simulink library "MickLibBlocks"  (R2014a)
settings: Solver=ode45  StartTime=0.0  StopTime=10.0  RelTol=1e-3
values from neighbouring files (symbols this model uses):
  a = param.a    [DSC_Control_Analysis.m]    (also in DSC_Control_Analysis_Exp.m; DSC_Speed_Control_Analysis.m; EmpiricalTireCurves.m = 1.35; FFW_Fx.m = sqrt(curvature/(2*clothoidLength)))
  b = 1.15    [EmpiricalTireCurves.m]
  Cf = param.fl.C + param.fr.C    [Fyf_lookup_table.m]
  FFWax = fliplr(ax)    [FFW_Fx.m]
  m = 1724    [EmpiricalTireCurves.m]
  max_axRegen = -90*2*.91*5.5/.32/m    [FFW_Fx.m]
  maxUxRegen = max(UxRegen)    [FFW_Fx.m]
  s = 0:Step:round(sMax/Step)*Step    [FFW_Fx.m]
  Ts = 0.002    [DSC_Control_Analysis.m]    (also in DSC_Control_Analysis_Exp.m; DSC_Speed_Control_Analysis.m; EC_params_nissan.m; Ext_MPCPara.m = SSD.Ts)
  UxConstant = sqrt(mu*trackRadius*g)    [FFW_Fx.m]
undefined symbols (not defined in the file or in its folder): alphaFrontLimit, alphaRearLimit, Cr, filtera, filterb, gain_force_psi, gainFrontAlphaSlip, gainRearAlphaSlip, gainRearKappaSlip, gainRearNoneSlip, kappaFrontLimit, kappaRearLimit, lkparams, numberFIR_force, param, psi_threshold, sr, steering_limit, wc
libraries: UserBlocks x6, simulink_need_slupdate x3, MickLibBlocks x2
(part 1 of 2)
settings Model: Creator=ddl  LastModifiedBy=cbeal

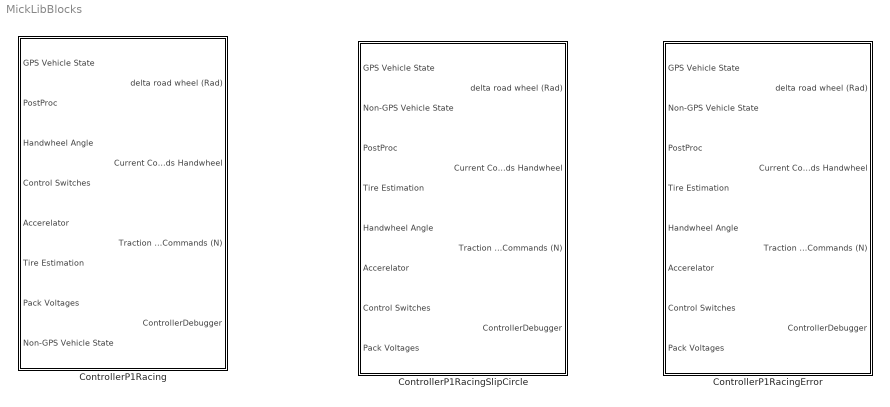
== system MickLibBlocks ==
  ControllerP1Racing : Subsystem
      mask init:
      | p1_params
  ControllerP1RacingError : Subsystem
      mask init:
      | p1_params
  ControllerP1RacingSlipCircle : Subsystem
      mask init:
      | p1_params

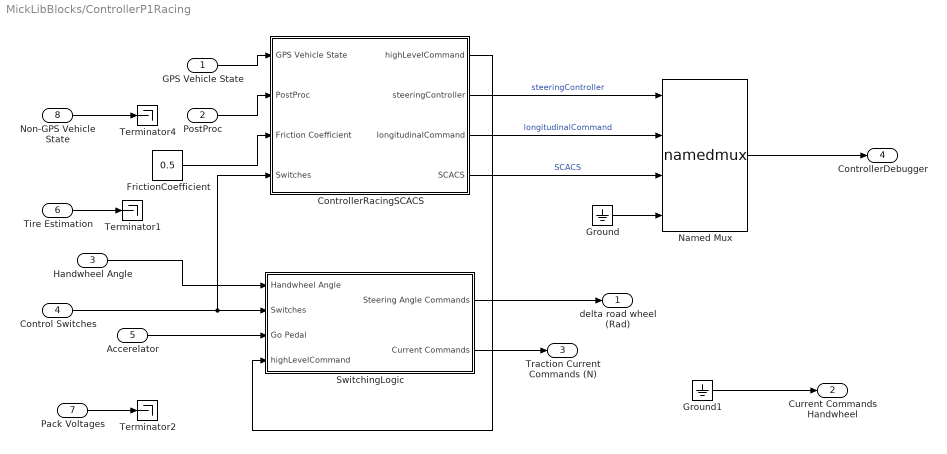
== system MickLibBlocks/ControllerP1Racing ==
  GPS Vehicle State : Inport
  PostProc : Inport  Port=2
  Handwheel Angle : Inport  Port=3
  Control Switches : Inport  Port=4
  Accerelator : Inport  Port=5
  Tire Estimation : Inport  Port=6
  Pack Voltages : Inport  Port=7
  Non-GPS Vehicle State : Inport  Port=8
  ControllerRacingSCACS : Subsystem
      mask init:
      | p1_params
  FrictionCoefficient : Constant  Value=0.5
  Ground : Ground
  Ground1 : Ground
  Named Mux : S-Function  FunctionName=namedmux  Parameters=inputcount,inputsizes  EnableBusSupport=off  mask{fname=datadescRacing}
      mask prompts: fname "Data description function name"
      mask help:
      | Combines input signals into a single output vector, according to a structure that provides the names and sizes of each signal.
      |
      | The parameter below should be set to the name of a function which returns a 1xN structure array, where N is the number of input signals.  The structure should contain fields "size" which specifies the width of the input signal, and "name" which specifies its name.
      mask init:
      | desc=eval(fname);
      | %if(class(desc)~='cell')
      | %	error('Incorrect description');
      | %end
      | inputcount=length(desc);
      | if((inputcount<1)|(inputcount>50))
      | 	error('Inappropriate number of inputs.');
      | end
      | 
      | inputsizes=[desc.size];
      | 
      | x=min(inputcount*ones(1,50),1:50);
      mask Display:
      | port_label('input',x(1),desc(x(1)).name);
      | port_label('input',x(2),desc(x(2)).name);
      | port_label('input',x(3),desc(x(3)).name);
      | port_label('input',x(4),desc(x(4)).name);
      | port_label('input',x(5),desc(x(5)).name);
      | port_label('input',x(6),desc(x(6)).name);
      | port_label('input',x(7),desc(x(7)).name);
      | port_label('input',x(8),desc(x(8)).name);
      | port_label('input',x(9),desc(x(9)).name);
      | port_label('input',x(10),desc(x(10)).name);
      | port_label('input',x(11),desc(x(11)).name);
      | port_label('input',x(12),desc(x(12)).name);
      | port_label('input',x(13),desc(x(13)).name);
      | port_label('input',x(14),desc(x(14)).name);
      | port_label('input',x(15),desc(x(15)).name);
      | port_label('input',x(16),desc(x(16)).name);
      | port_label('input',x(17),desc(x(17)).name);
      | port_label('input',x(18),desc(x(18)).name);
      | port_label('input',x(19),desc(x(19)).name);
      | port_label('input',x(20),desc(x(20)).name);
      | port_label('input',x(21),desc(x(21)).name);
      | port_label('input',x(22),desc(x(22)).name);
      | port_label('input',x(23),desc(x(23)).name);
      | port_label('input',x(24),desc(x(24)).name);
      | port_label('input',x(25),desc(x(25)).name);
      | port_label('input',x(26),desc(x(26)).name);
      | port_label('input',x(27),desc(x(27)).name);
      | port_label('input',x(28),desc(x(28)).name);
      | port_label('input',x(29),desc(x(29)).name);
      | port_label('input',x(30),desc(x(30)).name);
  SwitchingLogic : Subsystem
      mask init:
      | p1_params;
      | SteeringController;
  Terminator1 : Terminator
  Terminator2 : Terminator
  Terminator4 : Terminator
  delta road wheel (Rad) : Outport
  Current Commands Handwheel : Outport  Port=2
  Traction Current Commands (N) : Outport  Port=3
  ControllerDebugger : Outport  Port=4
  wires:
  Ground1/1 -> Current Commands Handwheel/1
  Named Mux/1 -> ControllerDebugger/1
  ControllerRacingSCACS/1(highLevelCommand) -> SwitchingLogic/4(highLevelCommand)
  GPS Vehicle State/1 -> ControllerRacingSCACS/1(GPS Vehicle State)
  PostProc/1 -> ControllerRacingSCACS/2(PostProc)
  Handwheel Angle/1 -> SwitchingLogic/1(Handwheel Angle)
  Accerelator/1 -> SwitchingLogic/3(Go Pedal)
  Control Switches/1 -> ControllerRacingSCACS/4(Switches), SwitchingLogic/2(Switches)
  SwitchingLogic/1(Steering Angle Commands) -> delta road wheel (Rad)/1
  SwitchingLogic/2(Current Commands) -> Traction Current Commands (N)/1
  ControllerRacingSCACS/2(steeringController) -> Named Mux/1  "steeringController"
  ControllerRacingSCACS/3(longitudinalCommand) -> Named Mux/2  "longitudinalCommand"
  ControllerRacingSCACS/4(SCACS) -> Named Mux/3  "SCACS"
  Non-GPS Vehicle State/1 -> Terminator4/1
  Tire Estimation/1 -> Terminator1/1
  Pack Voltages/1 -> Terminator2/1
  FrictionCoefficient/1 -> ControllerRacingSCACS/3(Friction Coefficient)
  Ground/1 -> Named Mux/4

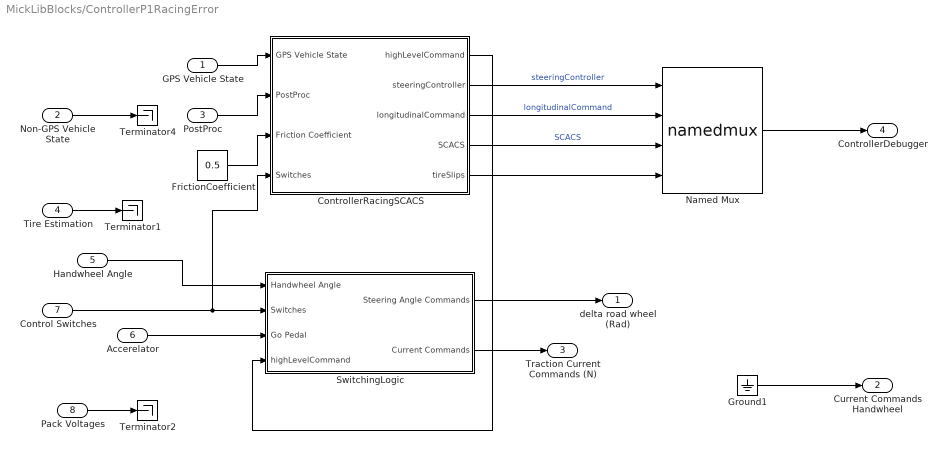
== system MickLibBlocks/ControllerP1RacingError ==
  GPS Vehicle State : Inport
  Non-GPS Vehicle State : Inport  Port=2
  PostProc : Inport  Port=3
  Tire Estimation : Inport  Port=4
  Handwheel Angle : Inport  Port=5
  Accerelator : Inport  Port=6
  Control Switches : Inport  Port=7
  Pack Voltages : Inport  Port=8
  ControllerRacingSCACS : Subsystem
      mask init:
      | p1_params
  FrictionCoefficient : Constant  Value=0.5
  Ground1 : Ground
  Named Mux : S-Function  FunctionName=namedmux  Parameters=inputcount,inputsizes  EnableBusSupport=off  mask{fname=datadescRacing}
      mask prompts: fname "Data description function name"
      mask help:
      | Combines input signals into a single output vector, according to a structure that provides the names and sizes of each signal.
      |
      | The parameter below should be set to the name of a function which returns a 1xN structure array, where N is the number of input signals.  The structure should contain fields "size" which specifies the width of the input signal, and "name" which specifies its name.
      mask init: same as MickLibBlocks/ControllerP1Racing/Named Mux
      mask Display:
      | port_label('input',x(1),desc(x(1)).name);
      | port_label('input',x(2),desc(x(2)).name);
      | port_label('input',x(3),desc(x(3)).name);
      | port_label('input',x(4),desc(x(4)).name);
      | port_label('input',x(5),desc(x(5)).name);
      | port_label('input',x(6),desc(x(6)).name);
      | port_label('input',x(7),desc(x(7)).name);
      | port_label('input',x(8),desc(x(8)).name);
      | port_label('input',x(9),desc(x(9)).name);
      | port_label('input',x(10),desc(x(10)).name);
      | port_label('input',x(11),desc(x(11)).name);
      | port_label('input',x(12),desc(x(12)).name);
      | port_label('input',x(13),desc(x(13)).name);
      | port_label('input',x(14),desc(x(14)).name);
      | port_label('input',x(15),desc(x(15)).name);
      | port_label('input',x(16),desc(x(16)).name);
      | port_label('input',x(17),desc(x(17)).name);
      | port_label('input',x(18),desc(x(18)).name);
      | port_label('input',x(19),desc(x(19)).name);
      | port_label('input',x(20),desc(x(20)).name);
      | port_label('input',x(21),desc(x(21)).name);
      | port_label('input',x(22),desc(x(22)).name);
      | port_label('input',x(23),desc(x(23)).name);
      | port_label('input',x(24),desc(x(24)).name);
      | port_label('input',x(25),desc(x(25)).name);
      | port_label('input',x(26),desc(x(26)).name);
      | port_label('input',x(27),desc(x(27)).name);
      | port_label('input',x(28),desc(x(28)).name);
      | port_label('input',x(29),desc(x(29)).name);
      | port_label('input',x(30),desc(x(30)).name);
  SwitchingLogic : Subsystem
      mask init:
      | p1_params;
      | SteeringController;
  Terminator1 : Terminator
  Terminator2 : Terminator
  Terminator4 : Terminator
  delta road wheel (Rad) : Outport
  Current Commands Handwheel : Outport  Port=2
  Traction Current Commands (N) : Outport  Port=3
  ControllerDebugger : Outport  Port=4
  wires:
  Ground1/1 -> Current Commands Handwheel/1
  FrictionCoefficient/1 -> ControllerRacingSCACS/3(Friction Coefficient)
  Pack Voltages/1 -> Terminator2/1
  Tire Estimation/1 -> Terminator1/1
  Non-GPS Vehicle State/1 -> Terminator4/1
  ControllerRacingSCACS/4(SCACS) -> Named Mux/3  "SCACS"
  ControllerRacingSCACS/3(longitudinalCommand) -> Named Mux/2  "longitudinalCommand"
  ControllerRacingSCACS/2(steeringController) -> Named Mux/1  "steeringController"
  SwitchingLogic/2(Current Commands) -> Traction Current Commands (N)/1
  SwitchingLogic/1(Steering Angle Commands) -> delta road wheel (Rad)/1
  Control Switches/1 -> SwitchingLogic/2(Switches), ControllerRacingSCACS/4(Switches)
  Accerelator/1 -> SwitchingLogic/3(Go Pedal)
  Handwheel Angle/1 -> SwitchingLogic/1(Handwheel Angle)
  PostProc/1 -> ControllerRacingSCACS/2(PostProc)
  GPS Vehicle State/1 -> ControllerRacingSCACS/1(GPS Vehicle State)
  ControllerRacingSCACS/1(highLevelCommand) -> SwitchingLogic/4(highLevelCommand)
  Named Mux/1 -> ControllerDebugger/1
  ControllerRacingSCACS/5(tireSlips) -> Named Mux/4

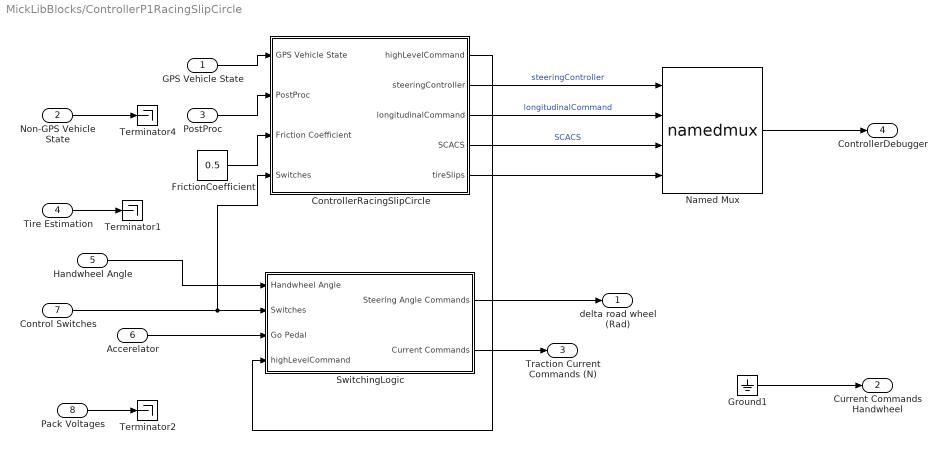
== system MickLibBlocks/ControllerP1RacingSlipCircle ==
  GPS Vehicle State : Inport
  Non-GPS Vehicle State : Inport  Port=2
  PostProc : Inport  Port=3
  Tire Estimation : Inport  Port=4
  Handwheel Angle : Inport  Port=5
  Accerelator : Inport  Port=6
  Control Switches : Inport  Port=7
  Pack Voltages : Inport  Port=8
  ControllerRacingSlipCircle : Subsystem
      mask init:
      | p1_params
  FrictionCoefficient : Constant  Value=0.5
  Ground1 : Ground
  Named Mux : S-Function  FunctionName=namedmux  Parameters=inputcount,inputsizes  EnableBusSupport=off  mask{fname=datadescRacing}
      mask prompts: fname "Data description function name"
      mask help:
      | Combines input signals into a single output vector, according to a structure that provides the names and sizes of each signal.
      |
      | The parameter below should be set to the name of a function which returns a 1xN structure array, where N is the number of input signals.  The structure should contain fields "size" which specifies the width of the input signal, and "name" which specifies its name.
      mask init: same as MickLibBlocks/ControllerP1Racing/Named Mux
      mask Display:
      | port_label('input',x(1),desc(x(1)).name);
      | port_label('input',x(2),desc(x(2)).name);
      | port_label('input',x(3),desc(x(3)).name);
      | port_label('input',x(4),desc(x(4)).name);
      | port_label('input',x(5),desc(x(5)).name);
      | port_label('input',x(6),desc(x(6)).name);
      | port_label('input',x(7),desc(x(7)).name);
      | port_label('input',x(8),desc(x(8)).name);
      | port_label('input',x(9),desc(x(9)).name);
      | port_label('input',x(10),desc(x(10)).name);
      | port_label('input',x(11),desc(x(11)).name);
      | port_label('input',x(12),desc(x(12)).name);
      | port_label('input',x(13),desc(x(13)).name);
      | port_label('input',x(14),desc(x(14)).name);
      | port_label('input',x(15),desc(x(15)).name);
      | port_label('input',x(16),desc(x(16)).name);
      | port_label('input',x(17),desc(x(17)).name);
      | port_label('input',x(18),desc(x(18)).name);
      | port_label('input',x(19),desc(x(19)).name);
      | port_label('input',x(20),desc(x(20)).name);
      | port_label('input',x(21),desc(x(21)).name);
      | port_label('input',x(22),desc(x(22)).name);
      | port_label('input',x(23),desc(x(23)).name);
      | port_label('input',x(24),desc(x(24)).name);
      | port_label('input',x(25),desc(x(25)).name);
      | port_label('input',x(26),desc(x(26)).name);
      | port_label('input',x(27),desc(x(27)).name);
      | port_label('input',x(28),desc(x(28)).name);
      | port_label('input',x(29),desc(x(29)).name);
      | port_label('input',x(30),desc(x(30)).name);
  SwitchingLogic : Subsystem
      mask init:
      | p1_params;
      | SteeringController;
  Terminator1 : Terminator
  Terminator2 : Terminator
  Terminator4 : Terminator
  delta road wheel (Rad) : Outport
  Current Commands Handwheel : Outport  Port=2
  Traction Current Commands (N) : Outport  Port=3
  ControllerDebugger : Outport  Port=4
  wires:
  ControllerRacingSlipCircle/5(tireSlips) -> Named Mux/4
  Named Mux/1 -> ControllerDebugger/1
  ControllerRacingSlipCircle/1(highLevelCommand) -> SwitchingLogic/4(highLevelCommand)
  GPS Vehicle State/1 -> ControllerRacingSlipCircle/1(GPS Vehicle State)
  PostProc/1 -> ControllerRacingSlipCircle/2(PostProc)
  Handwheel Angle/1 -> SwitchingLogic/1(Handwheel Angle)
  Accerelator/1 -> SwitchingLogic/3(Go Pedal)
  Control Switches/1 -> SwitchingLogic/2(Switches), ControllerRacingSlipCircle/4(Switches)
  SwitchingLogic/1(Steering Angle Commands) -> delta road wheel (Rad)/1
  SwitchingLogic/2(Current Commands) -> Traction Current Commands (N)/1
  ControllerRacingSlipCircle/2(steeringController) -> Named Mux/1  "steeringController"
  ControllerRacingSlipCircle/3(longitudinalCommand) -> Named Mux/2  "longitudinalCommand"
  ControllerRacingSlipCircle/4(SCACS) -> Named Mux/3  "SCACS"
  Non-GPS Vehicle State/1 -> Terminator4/1
  Tire Estimation/1 -> Terminator1/1
  Pack Voltages/1 -> Terminator2/1
  FrictionCoefficient/1 -> ControllerRacingSlipCircle/3(Friction Coefficient)
  Ground1/1 -> Current Commands Handwheel/1

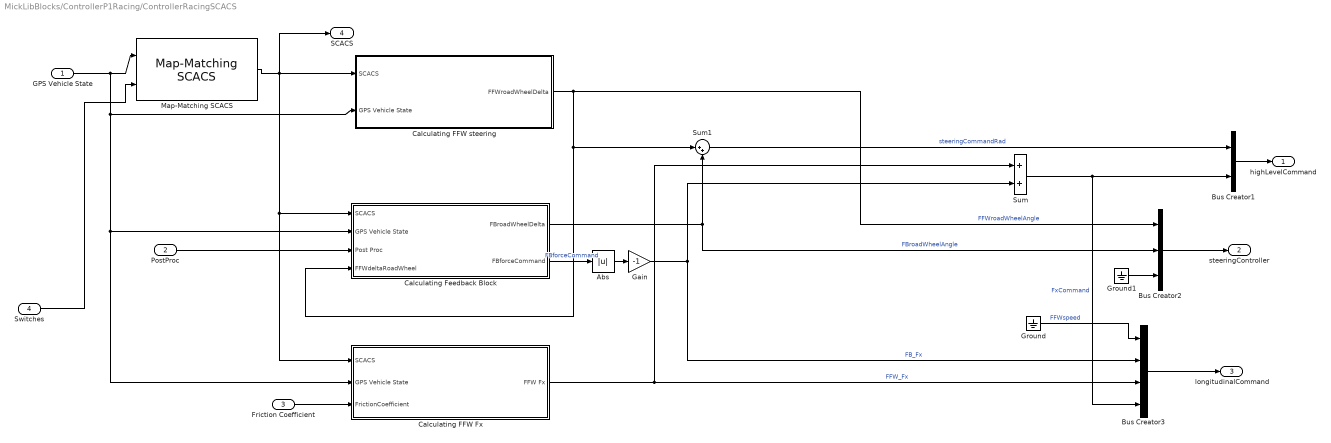
== system MickLibBlocks/ControllerP1Racing/ControllerRacingSCACS ==
  GPS Vehicle State : Inport
  PostProc : Inport  Port=2
  Friction Coefficient : Inport  Port=3
  Switches : Inport  Port=4
  Abs : Abs
  Bus Creator1 : BusCreator  Inputs=2
  Bus Creator2 : BusCreator  Inputs=3
  Bus Creator3 : BusCreator
  Calculating FFW Fx : Subsystem  TreatAsAtomicUnit=on
      mask init:
      | p1_params
      | FFW_Fx
  Calculating FFW steering : Subsystem  TreatAsAtomicUnit=on
  Calculating Feedback Block : Subsystem  TreatAsAtomicUnit=on
  Gain : Gain  Gain=-1  SampleTime=Ts
  Ground : Ground
  Ground1 : Ground
  Map-Matching SCACS : UserBlocks/Map-Matching SCACS
  Sum : Sum  SampleTime=Ts
  Sum1 : Sum  Inputs=|++
  highLevelCommand : Outport
  steeringController : Outport  Port=2
  longitudinalCommand : Outport  Port=3
  SCACS : Outport  Port=4
  wires:
  Switches/1 -> Map-Matching SCACS/2
  Sum/1 -> Bus Creator1/2, Bus Creator3/4  "FxCommand"
  PostProc/1 -> Calculating Feedback Block/3(Post Proc)
  Bus Creator1/1 -> highLevelCommand/1
  Bus Creator2/1 -> steeringController/1
  Bus Creator3/1 -> longitudinalCommand/1
  GPS Vehicle State/1 -> Map-Matching SCACS/1, Calculating FFW steering/2(GPS Vehicle State), Calculating Feedback Block/2(GPS Vehicle State), Calculating FFW Fx/2(GPS Vehicle State)
  Map-Matching SCACS/1 -> Calculating FFW steering/1(SCACS), SCACS/1, Calculating Feedback Block/1(SCACS), Calculating FFW Fx/1(SCACS)
  Calculating FFW steering/1(FFWroadWheelDelta) -> Calculating Feedback Block/4(FFWdeltaRoadWheel), Sum1/1, Bus Creator2/1  "FFWroadWheelAngle"
  Calculating Feedback Block/2(FBforceCommand) -> Abs/1  "FBforceCommand"
  Calculating Feedback Block/1(FBroadWheelDelta) -> Sum1/2, Bus Creator2/2  "FBroadWheelAngle"
  Sum1/1 -> Bus Creator1/1  "steeringCommandRad"
  Calculating FFW Fx/1(FFW Fx) -> Sum/1, Bus Creator3/3  "FFW_Fx"
  Abs/1 -> Gain/1
  Gain/1 -> Sum/2, Bus Creator3/2  "FB_Fx"
  Friction Coefficient/1 -> Calculating FFW Fx/3(FrictionCoefficient)
  Ground/1 -> Bus Creator3/1  "FFWspeed"
  Ground1/1 -> Bus Creator2/3

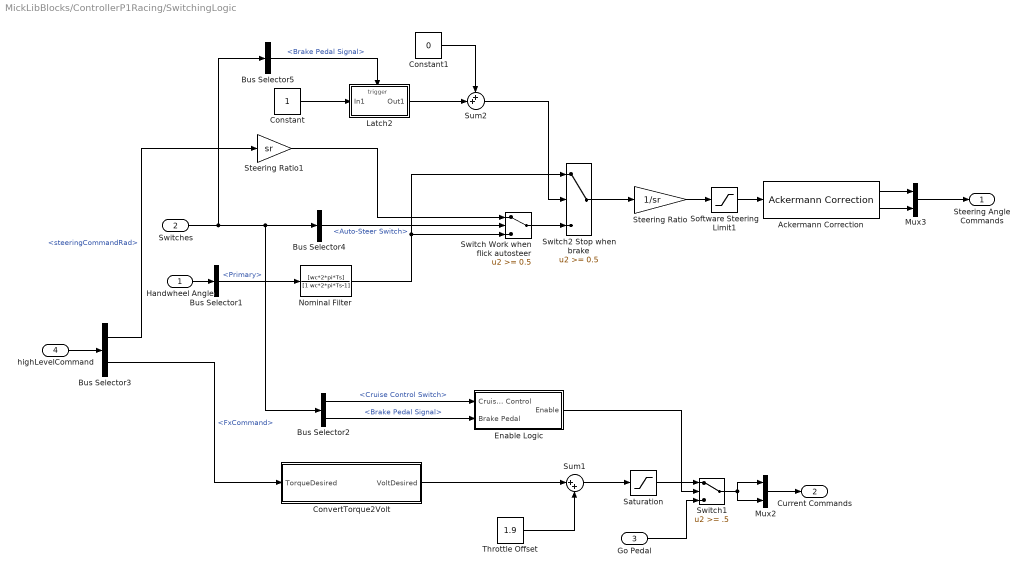
== system MickLibBlocks/ControllerP1Racing/SwitchingLogic ==
  Handwheel Angle : Inport
  Switches : Inport  Port=2
  Go Pedal : Inport  Port=3
  highLevelCommand : Inport  Port=4
  Ackermann Correction : UserBlocks/Steering Controller/Ackermann Correction
  Bus Selector1 : BusSelector  OutputSignals=Primary
  Bus Selector2 : BusSelector  OutputSignals=Cruise Control Switch,Brake Pedal Signal
  Bus Selector3 : BusSelector  OutputSignals=steeringCommandRad,FxCommand
  Bus Selector4 : BusSelector  OutputSignals=Auto-Steer Switch
  Bus Selector5 : BusSelector  OutputSignals=Brake Pedal Signal
  Constant : Constant  SampleTime=Ts
  Constant1 : Constant  Value=0  SampleTime=Ts
  ConvertTorque2Volt : Subsystem  TreatAsAtomicUnit=on
  Enable Logic : Subsystem
  Latch2 : Subsystem  TreatAsAtomicUnit=on
  Mux2 : Mux  Inputs=2
  Mux3 : Mux  Inputs=2
  Nominal Filter : DiscreteFilter  Numerator=[wc*2*pi*Ts]  Denominator=[1 wc*2*pi*Ts-1]  SampleTime=Ts
  Saturation : Saturate  UpperLimit=2.8  LowerLimit=.9
  Software Steering Limit1 : Saturate  UpperLimit=steering_limit*pi/180  LowerLimit=-steering_limit*pi/180
  Steering Ratio1 : Gain  Gain=sr  SaturateOnIntegerOverflow=on  OutDataTypeStr=Inherit: Same as input  ParamDataTypeStr=Inherit: Same as input
  Steering Ratio : Gain  Gain=1/sr  SaturateOnIntegerOverflow=on  OutDataTypeStr=Inherit: Same as input  ParamDataTypeStr=Inherit: Same as input
  Sum1 : Sum  Inputs=|++
  Sum2 : Sum  Inputs=++|
  Switch Work when flick autosteer : Switch  Threshold=0.5
  Switch1 : Switch  Threshold=.5
  Switch2 Stop when brake : Switch  Threshold=0.5  SampleTime=Ts
  Throttle Offset : Constant  Value=1.9
  Steering Angle Commands : Outport
  Current Commands : Outport  Port=2
  wires:
  highLevelCommand/1 -> Bus Selector3/1
  Handwheel Angle/1 -> Bus Selector1/1
  Switches/1 -> Bus Selector4/1, Bus Selector2/1, Bus Selector5/1
  Bus Selector4/1 -> Switch Work when flick autosteer/2  "<Auto-Steer Switch>"
  Bus Selector3/1 -> Steering Ratio1/1  "<steeringCommandRad>"
  Bus Selector1/1 -> Nominal Filter/1  "<Primary>"
  Nominal Filter/1 -> Switch Work when flick autosteer/3, Switch2 Stop when brake/1
  Steering Ratio/1 -> Software Steering Limit1/1
  Steering Ratio1/1 -> Switch Work when flick autosteer/1
  Bus Selector2/1 -> Enable Logic/1(Cruise Control)  "<Cruise Control Switch>"
  Bus Selector2/2 -> Enable Logic/2(Brake Pedal)  "<Brake Pedal Signal>"
  Go Pedal/1 -> Switch1/3
  ConvertTorque2Volt/1(VoltDesired) -> Sum1/1
  Throttle Offset/1 -> Sum1/2
  Saturation/1 -> Switch1/1
  Sum1/1 -> Saturation/1
  Mux2/1 -> Current Commands/1
  Switch1/1 -> Mux2/2, Mux2/1
  Bus Selector3/2 -> ConvertTorque2Volt/1(TorqueDesired)  "<FxCommand>"
  Enable Logic/1(Enable) -> Switch1/2
  Constant/1 -> Latch2/1(In1)
  Constant1/1 -> Sum2/1
  Switch Work when flick autosteer/1 -> Switch2 Stop when brake/3
  Switch2 Stop when brake/1 -> Steering Ratio/1
  Latch2/1(Out1) -> Sum2/2
  Sum2/1 -> Switch2 Stop when brake/2
  Bus Selector5/1 -> Latch2/Trigger  "<Brake Pedal Signal>"
  Mux3/1 -> Steering Angle Commands/1
  Software Steering Limit1/1 -> Ackermann Correction/1
  Ackermann Correction/1 -> Mux3/1
  Ackermann Correction/2 -> Mux3/2

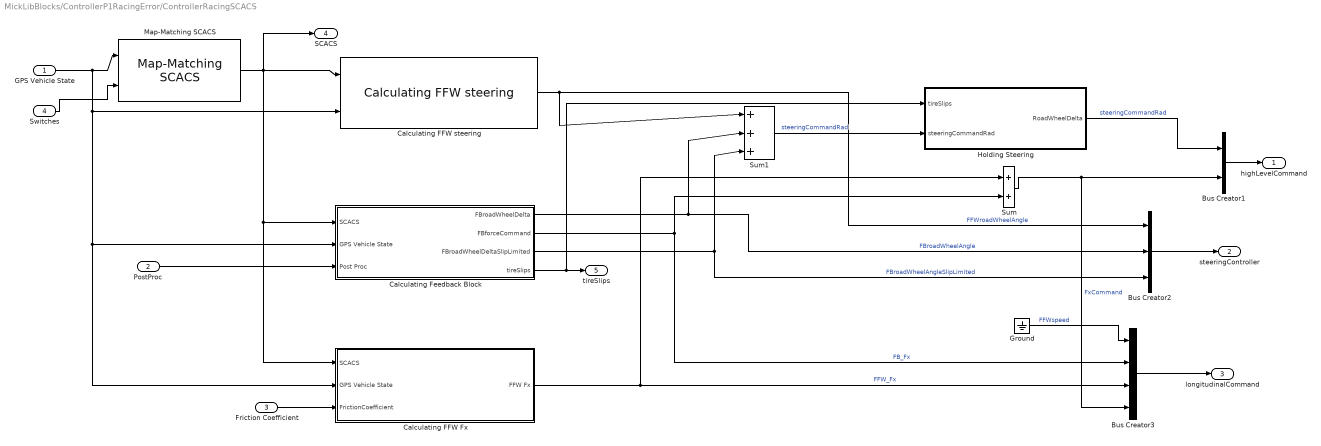
== system MickLibBlocks/ControllerP1RacingError/ControllerRacingSCACS ==
  GPS Vehicle State : Inport
  PostProc : Inport  Port=2
  Friction Coefficient : Inport  Port=3
  Switches : Inport  Port=4
  Bus Creator1 : BusCreator  Inputs=2
  Bus Creator2 : BusCreator  Inputs=3
  Bus Creator3 : BusCreator
  Calculating FFW Fx : Subsystem  TreatAsAtomicUnit=on
      mask init:
      | p1_params
      | FFW_Fx
  Calculating FFW steering : MickLibBlocks/ControllerP1Racing/ControllerRacingSCACS/Calculating FFW steering
  Calculating Feedback Block : Subsystem
  Ground : Ground
  Holding Steering : Subsystem
      mask init:
      | P1longitudinalController
  Map-Matching SCACS : UserBlocks/Map-Matching SCACS
  Sum : Sum  SampleTime=Ts
  Sum1 : Sum  Inputs=|+++  SampleTime=Ts
  highLevelCommand : Outport
  steeringController : Outport  Port=2
  longitudinalCommand : Outport  Port=3
  SCACS : Outport  Port=4
  tireSlips : Outport  Port=5
  wires:
  Ground/1 -> Bus Creator3/1  "FFWspeed"
  Friction Coefficient/1 -> Calculating FFW Fx/3(FrictionCoefficient)
  Calculating FFW Fx/1(FFW Fx) -> Bus Creator3/3, Sum/1  "FFW_Fx"
  Calculating Feedback Block/1(FBroadWheelDelta) -> Bus Creator2/2, Sum1/2  "FBroadWheelAngle"
  Calculating Feedback Block/2(FBforceCommand) -> Bus Creator3/2, Sum/2  "FB_Fx"
  Calculating FFW steering/1 -> Bus Creator2/1, Sum1/1  "FFWroadWheelAngle"
  Map-Matching SCACS/1 -> Calculating FFW Fx/1(SCACS), Calculating Feedback Block/1(SCACS), SCACS/1, Calculating FFW steering/1
  GPS Vehicle State/1 -> Calculating FFW Fx/2(GPS Vehicle State), Calculating Feedback Block/2(GPS Vehicle State), Calculating FFW steering/2, Map-Matching SCACS/1
  Bus Creator3/1 -> longitudinalCommand/1
  Bus Creator2/1 -> steeringController/1
  Bus Creator1/1 -> highLevelCommand/1
  PostProc/1 -> Calculating Feedback Block/3(Post Proc)
  Sum/1 -> Bus Creator3/4, Bus Creator1/2  "FxCommand"
  Calculating Feedback Block/3(FBroadWheelDeltaSlipLimited) -> Sum1/3, Bus Creator2/3  "FBroadWheelAngleSlipLimited"
  Calculating Feedback Block/4(tireSlips) -> tireSlips/1, Holding Steering/1(tireSlips)
  Sum1/1 -> Holding Steering/2(steeringCommandRad)  "steeringCommandRad"
  Holding Steering/1(RoadWheelDelta) -> Bus Creator1/1  "steeringCommandRad"
  Switches/1 -> Map-Matching SCACS/2

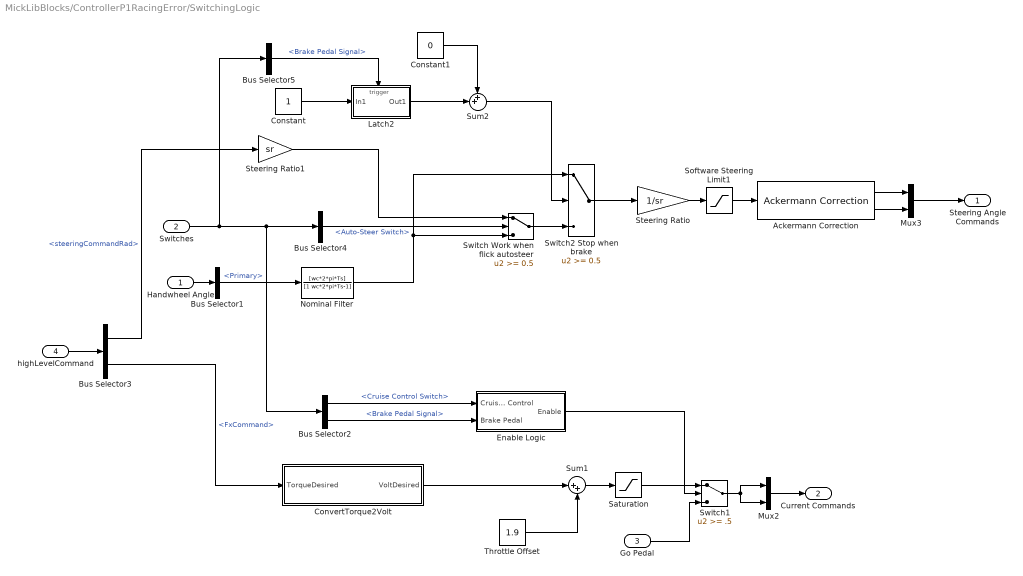
== system MickLibBlocks/ControllerP1RacingError/SwitchingLogic ==
  Handwheel Angle : Inport
  Switches : Inport  Port=2
  Go Pedal : Inport  Port=3
  highLevelCommand : Inport  Port=4
  Ackermann Correction : UserBlocks/Steering Controller/Ackermann Correction
  Bus Selector1 : BusSelector  OutputSignals=Primary
  Bus Selector2 : BusSelector  OutputSignals=Cruise Control Switch,Brake Pedal Signal
  Bus Selector3 : BusSelector  OutputSignals=steeringCommandRad,FxCommand
  Bus Selector4 : BusSelector  OutputSignals=Auto-Steer Switch
  Bus Selector5 : BusSelector  OutputSignals=Brake Pedal Signal
  Constant : Constant  SampleTime=Ts
  Constant1 : Constant  Value=0  SampleTime=Ts
  ConvertTorque2Volt : Subsystem  TreatAsAtomicUnit=on
  Enable Logic : Subsystem
  Latch2 : Subsystem  TreatAsAtomicUnit=on
  Mux2 : Mux  Inputs=2
  Mux3 : Mux  Inputs=2
  Nominal Filter : DiscreteFilter  Numerator=[wc*2*pi*Ts]  Denominator=[1 wc*2*pi*Ts-1]  SampleTime=Ts
  Saturation : Saturate  UpperLimit=2.8  LowerLimit=.9
  Software Steering Limit1 : Saturate  UpperLimit=steering_limit*pi/180  LowerLimit=-steering_limit*pi/180
  Steering Ratio1 : Gain  Gain=sr  SaturateOnIntegerOverflow=on  OutDataTypeStr=Inherit: Same as input  ParamDataTypeStr=Inherit: Same as input
  Steering Ratio : Gain  Gain=1/sr  SaturateOnIntegerOverflow=on  OutDataTypeStr=Inherit: Same as input  ParamDataTypeStr=Inherit: Same as input
  Sum1 : Sum  Inputs=|++
  Sum2 : Sum  Inputs=++|
  Switch Work when flick autosteer : Switch  Threshold=0.5
  Switch1 : Switch  Threshold=.5
  Switch2 Stop when brake : Switch  Threshold=0.5  SampleTime=Ts
  Throttle Offset : Constant  Value=1.9
  Steering Angle Commands : Outport
  Current Commands : Outport  Port=2
  wires:
  Saturation/1 -> Switch1/1
  Bus Selector5/1 -> Latch2/Trigger  "<Brake Pedal Signal>"
  Sum2/1 -> Switch2 Stop when brake/2
  Latch2/1(Out1) -> Sum2/2
  Switch2 Stop when brake/1 -> Steering Ratio/1
  Switch Work when flick autosteer/1 -> Switch2 Stop when brake/3
  Constant1/1 -> Sum2/1
  Constant/1 -> Latch2/1(In1)
  Enable Logic/1(Enable) -> Switch1/2
  Bus Selector3/2 -> ConvertTorque2Volt/1(TorqueDesired)  "<FxCommand>"
  Switch1/1 -> Mux2/1, Mux2/2
  Mux2/1 -> Current Commands/1
  Sum1/1 -> Saturation/1
  Throttle Offset/1 -> Sum1/2
  ConvertTorque2Volt/1(VoltDesired) -> Sum1/1
  Go Pedal/1 -> Switch1/3
  Bus Selector2/2 -> Enable Logic/2(Brake Pedal)  "<Brake Pedal Signal>"
  Bus Selector2/1 -> Enable Logic/1(Cruise Control)  "<Cruise Control Switch>"
  Steering Ratio1/1 -> Switch Work when flick autosteer/1
  Nominal Filter/1 -> Switch2 Stop when brake/1, Switch Work when flick autosteer/3
  Bus Selector1/1 -> Nominal Filter/1  "<Primary>"
  Bus Selector3/1 -> Steering Ratio1/1  "<steeringCommandRad>"
  Bus Selector4/1 -> Switch Work when flick autosteer/2  "<Auto-Steer Switch>"
  Switches/1 -> Bus Selector5/1, Bus Selector2/1, Bus Selector4/1
  Handwheel Angle/1 -> Bus Selector1/1
  highLevelCommand/1 -> Bus Selector3/1
  Mux3/1 -> Steering Angle Commands/1
  Software Steering Limit1/1 -> Ackermann Correction/1
  Ackermann Correction/1 -> Mux3/1
  Ackermann Correction/2 -> Mux3/2
  Steering Ratio/1 -> Software Steering Limit1/1

== system MickLibBlocks/ControllerP1RacingSlipCircle/ControllerRacingSlipCircle ==
  GPS Vehicle State : Inport
  PostProc : Inport  Port=2
  Friction Coefficient : Inport  Port=3
  Switches : Inport  Port=4
  Bus Creator1 : BusCreator  Inputs=2
  Bus Creator2 : BusCreator  Inputs=3
  Bus Creator3 : BusCreator
  Calculating FFW Fx : Subsystem  TreatAsAtomicUnit=on
      mask init:
      | p1_params
      | FFW_Fx
  Calculating FFW steering : MickLibBlocks/ControllerP1Racing/ControllerRacingSCACS/Calculating FFW steering
  Calculating Feedback Block : Subsystem
  Ground : Ground
  Map-Matching SCACS : UserBlocks/Map-Matching SCACS
  Sum : Sum  SampleTime=Ts
  Sum1 : Sum  Inputs=|+++  SampleTime=Ts
  highLevelCommand : Outport
  steeringController : Outport  Port=2
  longitudinalCommand : Outport  Port=3
  SCACS : Outport  Port=4
  tireSlips : Outport  Port=5
  wires:
  Calculating Feedback Block/4(tireSlips) -> tireSlips/1
  Calculating Feedback Block/3(FBroadWheelDeltaSlipLimited) -> Bus Creator2/3, Sum1/3  "FBroadWheelAngleSlipLimited"
  Sum/1 -> Bus Creator1/2, Bus Creator3/4  "FxCommand"
  PostProc/1 -> Calculating Feedback Block/3(Post Proc)
  Bus Creator1/1 -> highLevelCommand/1
  Bus Creator2/1 -> steeringController/1
  Bus Creator3/1 -> longitudinalCommand/1
  GPS Vehicle State/1 -> Calculating Feedback Block/2(GPS Vehicle State), Calculating FFW Fx/2(GPS Vehicle State), Calculating FFW steering/2, Map-Matching SCACS/1
  Map-Matching SCACS/1 -> SCACS/1, Calculating Feedback Block/1(SCACS), Calculating FFW Fx/1(SCACS), Calculating FFW steering/1
  Calculating FFW steering/1 -> Sum1/1, Bus Creator2/1  "FFWroadWheelAngle"
  Calculating Feedback Block/2(FBforceCommand) -> Sum/2, Bus Creator3/2  "FB_Fx"
  Calculating Feedback Block/1(FBroadWheelDelta) -> Sum1/2, Bus Creator2/2  "FBroadWheelAngle"
  Sum1/1 -> Bus Creator1/1  "steeringCommandRad"
  Calculating FFW Fx/1(FFW Fx) -> Sum/1, Bus Creator3/3  "FFW_Fx"
  Friction Coefficient/1 -> Calculating FFW Fx/3(FrictionCoefficient)
  Ground/1 -> Bus Creator3/1  "FFWspeed"
  Switches/1 -> Map-Matching SCACS/2

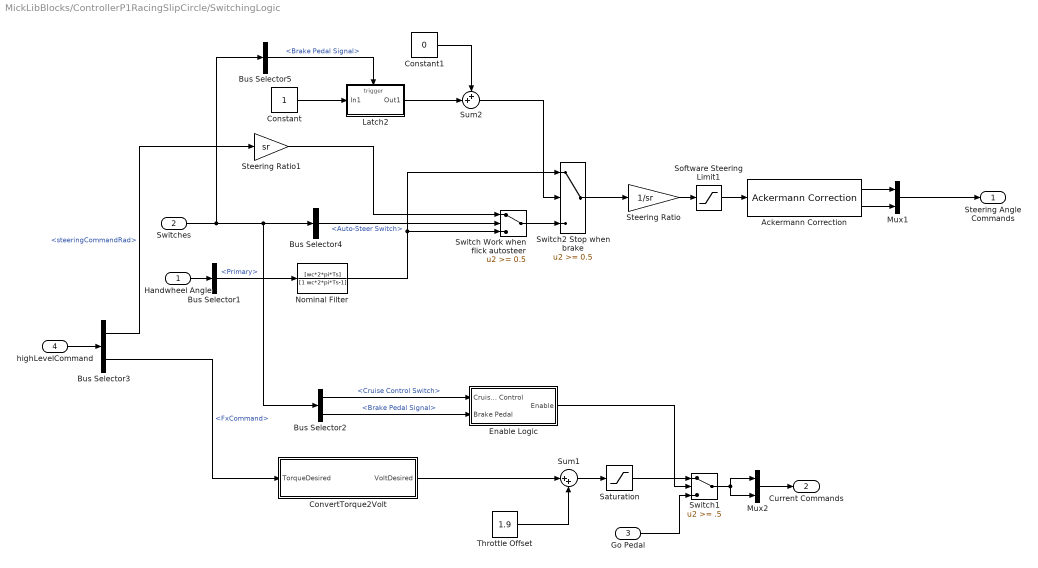
== system MickLibBlocks/ControllerP1RacingSlipCircle/SwitchingLogic ==
  Handwheel Angle : Inport
  Switches : Inport  Port=2
  Go Pedal : Inport  Port=3
  highLevelCommand : Inport  Port=4
  Ackermann Correction : UserBlocks/Steering Controller/Ackermann Correction
  Bus Selector1 : BusSelector  OutputSignals=Primary
  Bus Selector2 : BusSelector  OutputSignals=Cruise Control Switch,Brake Pedal Signal
  Bus Selector3 : BusSelector  OutputSignals=steeringCommandRad,FxCommand
  Bus Selector4 : BusSelector  OutputSignals=Auto-Steer Switch
  Bus Selector5 : BusSelector  OutputSignals=Brake Pedal Signal
  Constant : Constant  SampleTime=Ts
  Constant1 : Constant  Value=0  SampleTime=Ts
  ConvertTorque2Volt : Subsystem  TreatAsAtomicUnit=on
  Enable Logic : Subsystem
  Latch2 : Subsystem  TreatAsAtomicUnit=on
  Mux1 : Mux  Inputs=2
  Mux2 : Mux  Inputs=2
  Nominal Filter : DiscreteFilter  Numerator=[wc*2*pi*Ts]  Denominator=[1 wc*2*pi*Ts-1]  SampleTime=Ts
  Saturation : Saturate  UpperLimit=2.8  LowerLimit=.9
  Software Steering Limit1 : Saturate  UpperLimit=steering_limit*pi/180  LowerLimit=-steering_limit*pi/180
  Steering Ratio1 : Gain  Gain=sr  SaturateOnIntegerOverflow=on  OutDataTypeStr=Inherit: Same as input  ParamDataTypeStr=Inherit: Same as input
  Steering Ratio : Gain  Gain=1/sr  SaturateOnIntegerOverflow=on  OutDataTypeStr=Inherit: Same as input  ParamDataTypeStr=Inherit: Same as input
  Sum1 : Sum  Inputs=|++
  Sum2 : Sum  Inputs=++|
  Switch Work when flick autosteer : Switch  Threshold=0.5
  Switch1 : Switch  Threshold=.5
  Switch2 Stop when brake : Switch  Threshold=0.5  SampleTime=Ts
  Throttle Offset : Constant  Value=1.9
  Steering Angle Commands : Outport
  Current Commands : Outport  Port=2
  wires:
  highLevelCommand/1 -> Bus Selector3/1
  Handwheel Angle/1 -> Bus Selector1/1
  Switches/1 -> Bus Selector4/1, Bus Selector2/1, Bus Selector5/1
  Bus Selector4/1 -> Switch Work when flick autosteer/2  "<Auto-Steer Switch>"
  Bus Selector3/1 -> Steering Ratio1/1  "<steeringCommandRad>"
  Bus Selector1/1 -> Nominal Filter/1  "<Primary>"
  Nominal Filter/1 -> Switch Work when flick autosteer/3, Switch2 Stop when brake/1
  Steering Ratio/1 -> Software Steering Limit1/1
  Mux1/1 -> Steering Angle Commands/1
  Steering Ratio1/1 -> Switch Work when flick autosteer/1
  Bus Selector2/1 -> Enable Logic/1(Cruise Control)  "<Cruise Control Switch>"
  Bus Selector2/2 -> Enable Logic/2(Brake Pedal)  "<Brake Pedal Signal>"
  Go Pedal/1 -> Switch1/3
  ConvertTorque2Volt/1(VoltDesired) -> Sum1/1
  Throttle Offset/1 -> Sum1/2
  Sum1/1 -> Saturation/1
  Mux2/1 -> Current Commands/1
  Switch1/1 -> Mux2/2, Mux2/1
  Bus Selector3/2 -> ConvertTorque2Volt/1(TorqueDesired)  "<FxCommand>"
  Enable Logic/1(Enable) -> Switch1/2
  Constant/1 -> Latch2/1(In1)
  Constant1/1 -> Sum2/1
  Switch Work when flick autosteer/1 -> Switch2 Stop when brake/3
  Switch2 Stop when brake/1 -> Steering Ratio/1
  Latch2/1(Out1) -> Sum2/2
  Sum2/1 -> Switch2 Stop when brake/2
  Bus Selector5/1 -> Latch2/Trigger  "<Brake Pedal Signal>"
  Saturation/1 -> Switch1/1
  Software Steering Limit1/1 -> Ackermann Correction/1
  Ackermann Correction/1 -> Mux1/1
  Ackermann Correction/2 -> Mux1/2

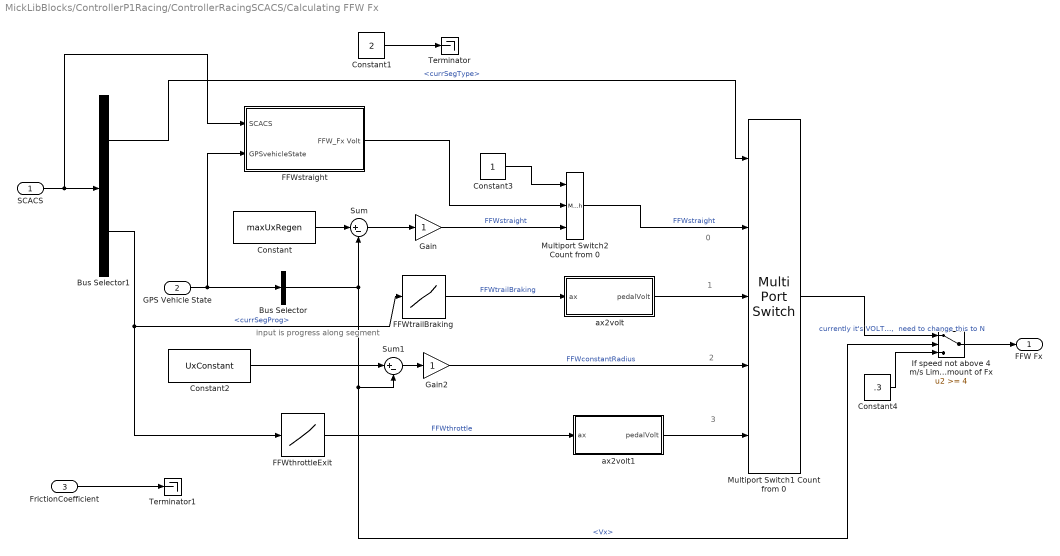
== system MickLibBlocks/ControllerP1Racing/ControllerRacingSCACS/Calculating FFW Fx ==
  note: input is progress along segment
  note: 0
  note: 1
  note: 2
  note: 3
  SCACS : Inport
  GPS Vehicle State : Inport  Port=2
  FrictionCoefficient : Inport  Port=3
  Bus Selector : BusSelector  OutputSignals=Vx
  Bus Selector1 : BusSelector  OutputSignals=currentOut.currSegType,currentOut.currSegProg
  Constant : Constant  Value=maxUxRegen  SampleTime=Ts
  Constant1 : Constant  Value=2  SampleTime=Ts
  Constant2 : Constant  Value=UxConstant  SampleTime=Ts
  Constant3 : Constant  SampleTime=Ts
  Constant4 : Constant  Value=.3  SampleTime=Ts
  FFWstraight : Subsystem
  FFWthrottleExit : Lookup  InputValues=s  Table=-fliplr(FFWax)  LookUpMeth=Interpolation-Use End Values  SampleTime=Ts
  FFWtrailBraking : Lookup  InputValues=s  Table=FFWax  LookUpMeth=Interpolation-Use End Values  SampleTime=Ts
  Gain : Gain  SampleTime=Ts
  Gain2 : Gain  SampleTime=Ts
  If speed not above 4 m/s Limit the amount of Fx : Switch  Threshold=4  SampleTime=Ts
  Multiport Switch1 Count from 0 : MultiPortSwitch  DataPortOrder=Zero-based contiguous  Inputs=4  zeroidx=on  SampleTime=Ts
  Multiport Switch2 Count from 0 : MultiPortSwitch  DataPortOrder=Zero-based contiguous  Inputs=2  zeroidx=on  SampleTime=Ts
  Sum : Sum  Inputs=|+-  SampleTime=Ts
  Sum1 : Sum  Inputs=|+-  SampleTime=Ts
  Terminator : Terminator
  Terminator1 : Terminator
  ax2volt : Subsystem
  ax2volt1 : Subsystem
  FFW Fx : Outport
  wires:
  SCACS/1 -> Bus Selector1/1, FFWstraight/1(SCACS)
  GPS Vehicle State/1 -> Bus Selector/1, FFWstraight/2(GPSvehicleState)
  Bus Selector/1 -> Sum/2, Sum1/2, If speed not above 4 m/s Limit the amount of Fx/2  "<Vx>"
  FFWtrailBraking/1 -> ax2volt/1(ax)  "FFWtrailBraking"
  FFWthrottleExit/1 -> ax2volt1/1(ax)  "FFWthrottle"
  Constant/1 -> Sum/1
  Sum/1 -> Gain/1
  Gain2/1 -> Multiport Switch1 Count from 0/4  "FFWconstantRadius"
  Constant2/1 -> Sum1/1
  Sum1/1 -> Gain2/1
  Bus Selector1/2 -> FFWtrailBraking/1, FFWthrottleExit/1  "<currSegProg>"
  ax2volt/1(pedalVolt) -> Multiport Switch1 Count from 0/3
  ax2volt1/1(pedalVolt) -> Multiport Switch1 Count from 0/5
  Constant1/1 -> Terminator/1
  Bus Selector1/1 -> Multiport Switch1 Count from 0/1  "<currSegType>"
  FFWstraight/1(FFW_Fx Volt) -> Multiport Switch2 Count from 0/2
  Multiport Switch2 Count from 0/1 -> Multiport Switch1 Count from 0/2  "FFWstraight"
  Gain/1 -> Multiport Switch2 Count from 0/3  "FFWstraight"
  Constant3/1 -> Multiport Switch2 Count from 0/1
  Constant4/1 -> If speed not above 4 m/s Limit the amount of Fx/3
  Multiport Switch1 Count from 0/1 -> If speed not above 4 m/s Limit the amount of Fx/1  "currently it's VOLT,  need to change this to N"
  If speed not above 4 m/s Limit the amount of Fx/1 -> FFW Fx/1
  FrictionCoefficient/1 -> Terminator1/1

== system MickLibBlocks/ControllerP1Racing/ControllerRacingSCACS/Calculating FFW steering ==
  SCACS : Inport
  GPS Vehicle State : Inport  Port=2
  Bus Selector1 : BusSelector  OutputSignals=matchOut.curvature
  Bus Selector2 : BusSelector  OutputSignals=Vx
  Mux : Mux  Inputs=2
  S-Function : S-Function  FunctionName=FFWcontrolClothoid  Parameters=Cf,Cr,m,a,b  EnableBusSupport=off
  FFWroadWheelDelta : Outport
  wires:
  Mux/1 -> S-Function/1
  Bus Selector2/1 -> Mux/2  "<Vx>"
  Bus Selector1/1 -> Mux/1  "<curvature>"
  GPS Vehicle State/1 -> Bus Selector2/1
  SCACS/1 -> Bus Selector1/1
  S-Function/1 -> FFWroadWheelDelta/1  "rad"

== system MickLibBlocks/ControllerP1Racing/ControllerRacingSCACS/Calculating Feedback Block ==
  SCACS : Inport
  GPS Vehicle State : Inport  Port=2
  Post Proc : Inport  Port=3
  FFWdeltaRoadWheel : Inport  Port=4
  Feedback Speed : Subsystem
      mask init:
      | p1_params
      | P1longitudinalController
  Feedback Steering Lane Keeping : Subsystem  TreatAsAtomicUnit=on
      mask init:
      | p1_params
      | lk_params
  FBroadWheelDelta : Outport
  FBforceCommand : Outport  Port=2
  wires:
  SCACS/1 -> Feedback Steering Lane Keeping/1(SCACS), Feedback Speed/4(SCACS)
  GPS Vehicle State/1 -> Feedback Speed/1(GPS Vehicle State)
  Feedback Steering Lane Keeping/1(FBroadWheelDelta) -> FBroadWheelDelta/1
  Post Proc/1 -> Feedback Speed/2(PostProc)
  FFWdeltaRoadWheel/1 -> Feedback Speed/3(FFWroadwheelDelta)
  Feedback Speed/1(torqueFBcommand) -> FBforceCommand/1

== system MickLibBlocks/ControllerP1Racing/SwitchingLogic/ConvertTorque2Volt ==
  TorqueDesired : Inport
  VoltDesired : Outport
  wires:
  TorqueDesired/1 -> VoltDesired/1

== system MickLibBlocks/ControllerP1Racing/SwitchingLogic/Enable Logic ==
  Cruise Control : Inport
  Brake Pedal : Inport  Port=2
  Delay : Subsystem
  Latch1 : Subsystem  TreatAsAtomicUnit=on
  Logical Operator : Logic  Operator=OR  AllPortsSameDT=off  OutDataTypeStr=float('double')
  Logical Operator1 : Logic  AllPortsSameDT=off  OutDataTypeStr=float('double')
  Logical Operator2 : Logic  Operator=NOT  AllPortsSameDT=off  OutDataTypeStr=float('double')
  Enable : Outport
  wires:
  Latch1/1(Out1) -> Enable/1
  Cruise Control/1 -> Delay/1(In), Logical Operator1/1
  Delay/1(Out) -> Logical Operator/1
  Brake Pedal/1 -> Logical Operator2/1, Logical Operator/2
  Logical Operator/1 -> Latch1/Trigger
  Logical Operator1/1 -> Latch1/1(In1)
  Logical Operator2/1 -> Logical Operator1/2

== system MickLibBlocks/ControllerP1Racing/SwitchingLogic/Latch2 ==
  In1 : Inport
  Trigger : TriggerPort
  Out1 : Outport  InitialOutput=0
  wires:
  In1/1 -> Out1/1

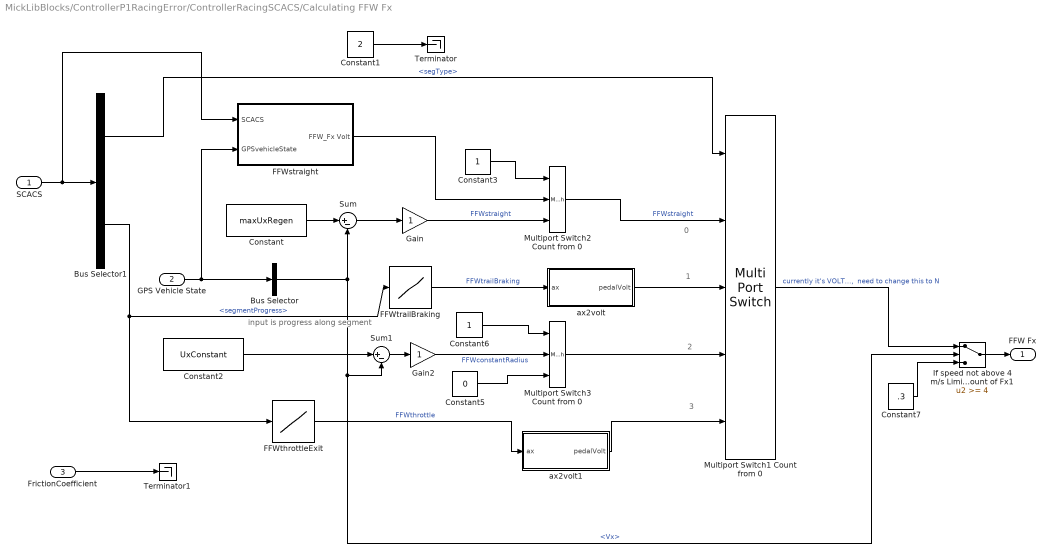
== system MickLibBlocks/ControllerP1RacingError/ControllerRacingSCACS/Calculating FFW Fx ==
  note: 3
  note: 2
  note: 1
  note: 0
  note: input is progress along segment
  SCACS : Inport
  GPS Vehicle State : Inport  Port=2
  FrictionCoefficient : Inport  Port=3
  Bus Selector : BusSelector  OutputSignals=Vx
  Bus Selector1 : BusSelector  OutputSignals=currentOut.segType,currentOut.segmentProgress
  Constant : Constant  Value=maxUxRegen  SampleTime=Ts
  Constant1 : Constant  Value=2  SampleTime=Ts
  Constant2 : Constant  Value=UxConstant  SampleTime=Ts
  Constant3 : Constant  SampleTime=Ts
  Constant5 : Constant  Value=0  SampleTime=Ts
  Constant6 : Constant  SampleTime=Ts
  Constant7 : Constant  Value=.3  SampleTime=Ts
  FFWstraight : Subsystem
  FFWthrottleExit : Lookup  InputValues=s  Table=-fliplr(FFWax)  LookUpMeth=Interpolation-Use End Values  SampleTime=Ts
  FFWtrailBraking : Lookup  InputValues=s  Table=FFWax  LookUpMeth=Interpolation-Use End Values  SampleTime=Ts
  Gain : Gain  SampleTime=Ts
  Gain2 : Gain  SampleTime=Ts
  If speed not above 4 m/s Limit the amount of Fx1 : Switch  Threshold=4  SampleTime=Ts
  Multiport Switch1 Count from 0 : MultiPortSwitch  DataPortOrder=Zero-based contiguous  Inputs=4  zeroidx=on  SampleTime=Ts
  Multiport Switch2 Count from 0 : MultiPortSwitch  DataPortOrder=Zero-based contiguous  Inputs=2  zeroidx=on  SampleTime=Ts
  Multiport Switch3 Count from 0 : MultiPortSwitch  DataPortOrder=Zero-based contiguous  Inputs=2  zeroidx=on  SampleTime=Ts
  Sum : Sum  Inputs=|+-  SampleTime=Ts
  Sum1 : Sum  Inputs=|+-  SampleTime=Ts
  Terminator : Terminator
  Terminator1 : Terminator
  ax2volt : Subsystem
  ax2volt1 : Subsystem
  FFW Fx : Outport
  wires:
  If speed not above 4 m/s Limit the amount of Fx1/1 -> FFW Fx/1
  Constant7/1 -> If speed not above 4 m/s Limit the amount of Fx1/3
  Multiport Switch1 Count from 0/1 -> If speed not above 4 m/s Limit the amount of Fx1/1  "currently it's VOLT,  need to change this to N"
  FrictionCoefficient/1 -> Terminator1/1
  Constant3/1 -> Multiport Switch2 Count from 0/1
  Gain/1 -> Multiport Switch2 Count from 0/3  "FFWstraight"
  Multiport Switch2 Count from 0/1 -> Multiport Switch1 Count from 0/2  "FFWstraight"
  FFWstraight/1(FFW_Fx Volt) -> Multiport Switch2 Count from 0/2
  Bus Selector1/1 -> Multiport Switch1 Count from 0/1  "<segType>"
  Constant1/1 -> Terminator/1
  ax2volt1/1(pedalVolt) -> Multiport Switch1 Count from 0/5
  ax2volt/1(pedalVolt) -> Multiport Switch1 Count from 0/3
  Bus Selector1/2 -> FFWthrottleExit/1, FFWtrailBraking/1  "<segmentProgress>"
  Sum1/1 -> Gain2/1
  Constant2/1 -> Sum1/1
  Sum/1 -> Gain/1
  Constant/1 -> Sum/1
  FFWthrottleExit/1 -> ax2volt1/1(ax)  "FFWthrottle"
  FFWtrailBraking/1 -> ax2volt/1(ax)  "FFWtrailBraking"
  Bus Selector/1 -> If speed not above 4 m/s Limit the amount of Fx1/2, Sum1/2, Sum/2  "<Vx>"
  GPS Vehicle State/1 -> FFWstraight/2(GPSvehicleState), Bus Selector/1
  SCACS/1 -> FFWstraight/1(SCACS), Bus Selector1/1
  Multiport Switch3 Count from 0/1 -> Multiport Switch1 Count from 0/4
  Gain2/1 -> Multiport Switch3 Count from 0/2  "FFWconstantRadius"
  Constant5/1 -> Multiport Switch3 Count from 0/3
  Constant6/1 -> Multiport Switch3 Count from 0/1

== system MickLibBlocks/ControllerP1RacingError/ControllerRacingSCACS/Calculating Feedback Block ==
  SCACS : Inport
  GPS Vehicle State : Inport  Port=2
  Post Proc : Inport  Port=3
  Constant : Constant  Value=0  SampleTime=Ts
  Feedback Fx : Subsystem
      mask init:
      | p1_params
      | P1longitudinalController
  Feedback Steering Lane Keeping : Subsystem  TreatAsAtomicUnit=on
      mask init:
      | p1_params
      | lk_params
  calculateSlips : Subsystem
      mask init:
      | p1_params
      | [filterb,filtera]=butter(5,0.02);
  FBroadWheelDelta : Outport
  FBforceCommand : Outport  Port=2
  FBroadWheelDeltaSlipLimited : Outport  Port=3
  tireSlips : Outport  Port=4
  wires:
  Feedback Fx/1(forceFBcommand) -> FBforceCommand/1
  Post Proc/1 -> calculateSlips/2(PostProc)
  Feedback Steering Lane Keeping/1(FBroadWheelDelta) -> FBroadWheelDelta/1
  GPS Vehicle State/1 -> Feedback Fx/1(GPS Vehicle State), calculateSlips/1(GPS Vehicle State)
  SCACS/1 -> Feedback Steering Lane Keeping/1(SCACS), Feedback Fx/4(SCACS)
  calculateSlips/1(tireSlips) -> tireSlips/1, Feedback Fx/2(tireSlips)
  Constant/1 -> FBroadWheelDeltaSlipLimited/1, Feedback Fx/3(FBroadWheelDeltaSlipLimited)

== system MickLibBlocks/ControllerP1RacingError/ControllerRacingSCACS/Holding Steering ==
  tireSlips : Inport
  steeringCommandRad : Inport  Port=2
  Bus Creator1 : BusCreator
  Constant : Constant  Value=alphaFrontLimit  SampleTime=Ts
  Constant1 : Constant  Value=alphaRearLimit  SampleTime=Ts
  Constant2 : Constant  Value=kappaFrontLimit  SampleTime=Ts
  Constant3 : Constant  Value=kappaRearLimit  SampleTime=Ts
  Integer Delay : Delay  DelayLength=1  InputProcessing=Inherited  SampleTime=Ts
  Mux : Mux
  S-Function3 : S-Function  FunctionName=holdingSteering  EnableBusSupport=off
  RoadWheelDelta : Outport
  wires:
  Integer Delay/1 -> Mux/3
  Bus Creator1/1 -> Mux/4
  Constant/1 -> Bus Creator1/1
  Constant1/1 -> Bus Creator1/2
  Constant2/1 -> Bus Creator1/3
  Constant3/1 -> Bus Creator1/4
  S-Function3/1 -> Integer Delay/1, RoadWheelDelta/1
  Mux/1 -> S-Function3/1
  steeringCommandRad/1 -> Mux/2
  tireSlips/1 -> Mux/1

== system MickLibBlocks/ControllerP1RacingError/SwitchingLogic/ConvertTorque2Volt ==
  TorqueDesired : Inport
  VoltDesired : Outport
  wires:
  TorqueDesired/1 -> VoltDesired/1

== system MickLibBlocks/ControllerP1RacingError/SwitchingLogic/Enable Logic ==
  Cruise Control : Inport
  Brake Pedal : Inport  Port=2
  Delay : Subsystem
  Latch1 : Subsystem  TreatAsAtomicUnit=on
  Logical Operator : Logic  Operator=OR  AllPortsSameDT=off  OutDataTypeStr=float('double')
  Logical Operator1 : Logic  AllPortsSameDT=off  OutDataTypeStr=float('double')
  Logical Operator2 : Logic  Operator=NOT  AllPortsSameDT=off  OutDataTypeStr=float('double')
  Enable : Outport
  wires:
  Logical Operator2/1 -> Logical Operator1/2
  Logical Operator1/1 -> Latch1/1(In1)
  Logical Operator/1 -> Latch1/Trigger
  Brake Pedal/1 -> Logical Operator/2, Logical Operator2/1
  Delay/1(Out) -> Logical Operator/1
  Cruise Control/1 -> Logical Operator1/1, Delay/1(In)
  Latch1/1(Out1) -> Enable/1

== system MickLibBlocks/ControllerP1RacingError/SwitchingLogic/Latch2 ==
  In1 : Inport
  Trigger : TriggerPort
  Out1 : Outport  InitialOutput=0
  wires:
  In1/1 -> Out1/1

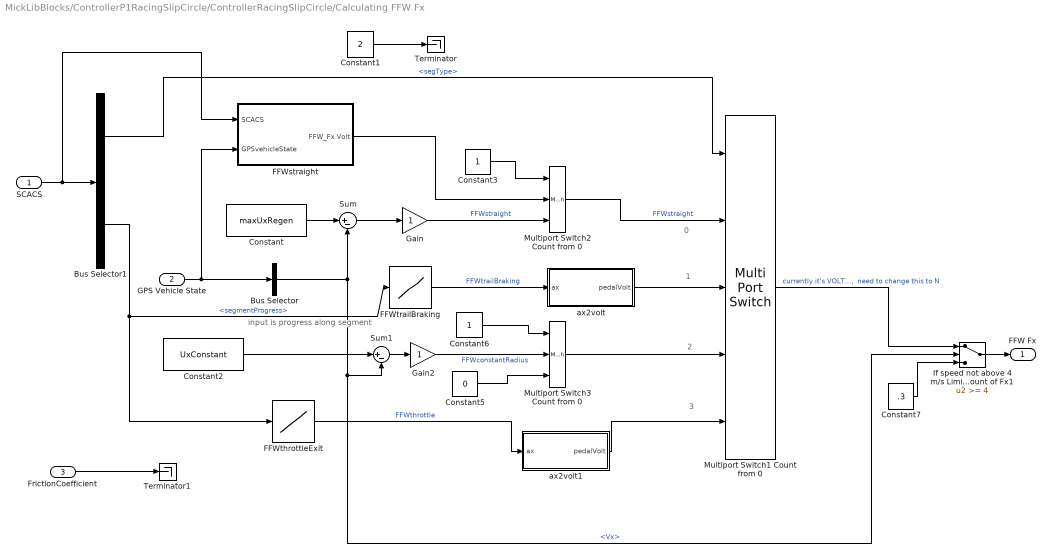
== system MickLibBlocks/ControllerP1RacingSlipCircle/ControllerRacingSlipCircle/Calculating FFW Fx ==
  note: input is progress along segment
  note: 0
  note: 1
  note: 2
  note: 3
  SCACS : Inport
  GPS Vehicle State : Inport  Port=2
  FrictionCoefficient : Inport  Port=3
  Bus Selector : BusSelector  OutputSignals=Vx
  Bus Selector1 : BusSelector  OutputSignals=currentOut.segType,currentOut.segmentProgress
  Constant : Constant  Value=maxUxRegen  SampleTime=Ts
  Constant1 : Constant  Value=2  SampleTime=Ts
  Constant2 : Constant  Value=UxConstant  SampleTime=Ts
  Constant3 : Constant  SampleTime=Ts
  Constant5 : Constant  Value=0  SampleTime=Ts
  Constant6 : Constant  SampleTime=Ts
  Constant7 : Constant  Value=.3  SampleTime=Ts
  FFWstraight : Subsystem
  FFWthrottleExit : Lookup  InputValues=s  Table=-fliplr(FFWax)  LookUpMeth=Interpolation-Use End Values  SampleTime=Ts
  FFWtrailBraking : Lookup  InputValues=s  Table=FFWax  LookUpMeth=Interpolation-Use End Values  SampleTime=Ts
  Gain : Gain  SampleTime=Ts
  Gain2 : Gain  SampleTime=Ts
  If speed not above 4 m/s Limit the amount of Fx1 : Switch  Threshold=4  SampleTime=Ts
  Multiport Switch1 Count from 0 : MultiPortSwitch  DataPortOrder=Zero-based contiguous  Inputs=4  zeroidx=on  SampleTime=Ts
  Multiport Switch2 Count from 0 : MultiPortSwitch  DataPortOrder=Zero-based contiguous  Inputs=2  zeroidx=on  SampleTime=Ts
  Multiport Switch3 Count from 0 : MultiPortSwitch  DataPortOrder=Zero-based contiguous  Inputs=2  zeroidx=on  SampleTime=Ts
  Sum : Sum  Inputs=|+-  SampleTime=Ts
  Sum1 : Sum  Inputs=|+-  SampleTime=Ts
  Terminator : Terminator
  Terminator1 : Terminator
  ax2volt : Subsystem
  ax2volt1 : Subsystem
  FFW Fx : Outport
  wires:
  Constant6/1 -> Multiport Switch3 Count from 0/1
  Constant5/1 -> Multiport Switch3 Count from 0/3
  Gain2/1 -> Multiport Switch3 Count from 0/2  "FFWconstantRadius"
  Multiport Switch3 Count from 0/1 -> Multiport Switch1 Count from 0/4
  SCACS/1 -> Bus Selector1/1, FFWstraight/1(SCACS)
  GPS Vehicle State/1 -> Bus Selector/1, FFWstraight/2(GPSvehicleState)
  Bus Selector/1 -> Sum/2, Sum1/2, If speed not above 4 m/s Limit the amount of Fx1/2  "<Vx>"
  FFWtrailBraking/1 -> ax2volt/1(ax)  "FFWtrailBraking"
  FFWthrottleExit/1 -> ax2volt1/1(ax)  "FFWthrottle"
  Constant/1 -> Sum/1
  Sum/1 -> Gain/1
  Constant2/1 -> Sum1/1
  Sum1/1 -> Gain2/1
  Bus Selector1/2 -> FFWtrailBraking/1, FFWthrottleExit/1  "<segmentProgress>"
  ax2volt/1(pedalVolt) -> Multiport Switch1 Count from 0/3
  ax2volt1/1(pedalVolt) -> Multiport Switch1 Count from 0/5
  Constant1/1 -> Terminator/1
  Bus Selector1/1 -> Multiport Switch1 Count from 0/1  "<segType>"
  FFWstraight/1(FFW_Fx Volt) -> Multiport Switch2 Count from 0/2
  Multiport Switch2 Count from 0/1 -> Multiport Switch1 Count from 0/2  "FFWstraight"
  Gain/1 -> Multiport Switch2 Count from 0/3  "FFWstraight"
  Constant3/1 -> Multiport Switch2 Count from 0/1
  FrictionCoefficient/1 -> Terminator1/1
  Multiport Switch1 Count from 0/1 -> If speed not above 4 m/s Limit the amount of Fx1/1  "currently it's VOLT,  need to change this to N"
  Constant7/1 -> If speed not above 4 m/s Limit the amount of Fx1/3
  If speed not above 4 m/s Limit the amount of Fx1/1 -> FFW Fx/1

== system MickLibBlocks/ControllerP1RacingSlipCircle/ControllerRacingSlipCircle/Calculating Feedback Block ==
  SCACS : Inport
  GPS Vehicle State : Inport  Port=2
  Post Proc : Inport  Port=3
  Feedback Fx : Subsystem
      mask init:
      | p1_params
      | P1longitudinalController
  Feedback Steering Lane Keeping : Subsystem  TreatAsAtomicUnit=on
      mask init:
      | p1_params
      | lk_params
  Feedback Steering Limit Slip : Subsystem  TreatAsAtomicUnit=on
      mask init:
      | p1_params
      | P1longitudinalController
  calculateSlips : Subsystem
      mask init:
      | p1_params
      | [filterb,filtera]=butter(5,0.02);
  FBroadWheelDelta : Outport
  FBforceCommand : Outport  Port=2
  FBroadWheelDeltaSlipLimited : Outport  Port=3
  tireSlips : Outport  Port=4
  wires:
  Feedback Steering Limit Slip/1(FBroadWheelDeltaSlipLimited) -> Feedback Fx/3(FBroadWheelDeltaSlipLimited), FBroadWheelDeltaSlipLimited/1
  calculateSlips/1(tireSlips) -> Feedback Fx/2(tireSlips), tireSlips/1, Feedback Steering Limit Slip/1(tireSlips)
  SCACS/1 -> Feedback Fx/4(SCACS), Feedback Steering Lane Keeping/1(SCACS)
  GPS Vehicle State/1 -> calculateSlips/1(GPS Vehicle State), Feedback Fx/1(GPS Vehicle State)
  Feedback Steering Lane Keeping/1(FBroadWheelDelta) -> FBroadWheelDelta/1
  Post Proc/1 -> calculateSlips/2(PostProc)
  Feedback Fx/1(forceFBcommand) -> FBforceCommand/1

== system MickLibBlocks/ControllerP1RacingSlipCircle/SwitchingLogic/ConvertTorque2Volt ==
  TorqueDesired : Inport
  VoltDesired : Outport
  wires:
  TorqueDesired/1 -> VoltDesired/1

== system MickLibBlocks/ControllerP1RacingSlipCircle/SwitchingLogic/Enable Logic ==
  Cruise Control : Inport
  Brake Pedal : Inport  Port=2
  Delay : Subsystem
  Latch1 : Subsystem  TreatAsAtomicUnit=on
  Logical Operator : Logic  Operator=OR  AllPortsSameDT=off  OutDataTypeStr=float('double')
  Logical Operator1 : Logic  AllPortsSameDT=off  OutDataTypeStr=float('double')
  Logical Operator2 : Logic  Operator=NOT  AllPortsSameDT=off  OutDataTypeStr=float('double')
  Enable : Outport
  wires:
  Latch1/1(Out1) -> Enable/1
  Cruise Control/1 -> Delay/1(In), Logical Operator1/1
  Delay/1(Out) -> Logical Operator/1
  Brake Pedal/1 -> Logical Operator2/1, Logical Operator/2
  Logical Operator/1 -> Latch1/Trigger
  Logical Operator1/1 -> Latch1/1(In1)
  Logical Operator2/1 -> Logical Operator1/2

== system MickLibBlocks/ControllerP1RacingSlipCircle/SwitchingLogic/Latch2 ==
  In1 : Inport
  Trigger : TriggerPort
  Out1 : Outport  InitialOutput=0
  wires:
  In1/1 -> Out1/1

== system MickLibBlocks/ControllerP1Racing/ControllerRacingSCACS/Calculating FFW Fx/FFWstraight ==
  SCACS : Inport
  GPSvehicleState : Inport  Port=2
  Bus Selector : BusSelector  OutputSignals=Vx
  Bus Selector1 : BusSelector  OutputSignals=currentOut.distToNxtSeg,currentOut.currSegType
  Mux : Mux  Inputs=3
  S-Function3 : S-Function  FunctionName=FFWstraight  Parameters=max_axRegen,maxUxRegen  EnableBusSupport=off
  FFW_Fx Volt : Outport
  wires:
  GPSvehicleState/1 -> Bus Selector/1
  S-Function3/1 -> FFW_Fx Volt/1
  SCACS/1 -> Bus Selector1/1
  Mux/1 -> S-Function3/1
  Bus Selector/1 -> Mux/1  "<Vx>"
  Bus Selector1/1 -> Mux/2  "<distToNxtSeg>"
  Bus Selector1/2 -> Mux/3  "<currSegType>"

== system MickLibBlocks/ControllerP1Racing/ControllerRacingSCACS/Calculating FFW Fx/ax2volt ==
  ax : Inport
  Constant : Constant  Value=1.9  SampleTime=Ts
  Gear Ratio : Gain  Gain=1/5.5  SampleTime=Ts
  Sum : Sum  Inputs=|+-
  Torque2volt : Lookup  InputValues=[-90,0,210]  Table=[0,1.9,2.8]  LookUpMeth=Interpolation-Use End Values  SampleTime=Ts
  convert to force : Gain  Gain=m  SampleTime=Ts
  motor efficiency : Gain  Gain=1/.91  SampleTime=Ts
  "two motors " : Gain  Gain=1/2  SampleTime=Ts
  wheel radius : Gain  Gain=.32  SampleTime=Ts
  pedalVolt : Outport
  wires:
  ax/1 -> convert to force/1
  convert to force/1 -> wheel radius/1  "force required"
  wheel radius/1 -> Gear Ratio/1  "torque required @ wheelS"
  Gear Ratio/1 -> motor efficiency/1
  motor efficiency/1 -> "two motors "/1  "torque required  @ motorS"
  "two motors "/1 -> Torque2volt/1  "torque required  @ each motor"
  Torque2volt/1 -> Sum/1
  Sum/1 -> pedalVolt/1
  Constant/1 -> Sum/2  "remove offset as this offset will be add later in the switching logic block"
